simulink library "bcm"  (R2021b)
settings: Solver=VariableStepAuto  StartTime=0.0  StopTime=10.0  RelTol=1e-3
undefined symbols (not defined in the file or in its folder): KBCM_ShowUPT_cnt
libraries: simulink x33
(part 2 of 2)

== stateflow chart bcm/BCM/BCM/ExteriorLight/Chart1 ==
  state FollowMeSW [parallel]
    settings: executionOrder=1
    state sRelease
    state sPress
    (default) -> sRelease
    sRelease -> sPress : [VINP_FollowMeSW_flg==1]/{AutoCut.eFollow;}
    sPress -> sRelease : [VINP_FollowMeSW_flg==0]
  state RFogLamp [parallel]
    settings: executionOrder=2
    state sON
      en:VBCM_RrFogLamp_flg=1;
    state sOFF
      en:VBCM_RrFogLamp_flg=0;
    (default) -> RFogLamp.sOFF
    RFogLamp.sOFF -> RFogLamp.sON : [VPMM_PwrSta_enum>3&&....
        | VINP_RFogLampSW_flg==1&&....
        | VBCM_LBeam_flg==1]
    RFogLamp.sON -> RFogLamp.sOFF : [VPMM_PwrSta_enum<=3||....
        | VINP_RFogLampSW_flg==0||....
        | VBCM_LBeam_flg==0]
  state DRL [parallel]
    settings: executionOrder=3
    state sOFF
      en:VBCM_LDRL_flg=0;
      VBCM_RDRL_flg=0;
    state DRL_Opearting
      state sDebounce
      state sON
        en:VBCM_LDRL_flg=1;
        VBCM_RDRL_flg=1;
      note: 300 ms
      state TurnLeft
        en:VBCM_LDRL_flg=0;
        VBCM_RDRL_flg=1;
      state TurnRight
        en:VBCM_LDRL_flg=1;
        VBCM_RDRL_flg=0;
      sDebounce -> (junction 119) : [after(30,tick)]
      (junction 119) -> DRL.DRL_Opearting.sON [order 1] : [VBCM_OutMode_enum==0]
      (junction 119) -> (junction 120) [order 2]
      DRL.DRL_Opearting.sON -> TurnLeft [order 1] : [VBCM_OutMode_enum==1]
      TurnLeft -> DRL.DRL_Opearting.sON [order 1] : [VBCM_OutMode_enum==0]
      TurnRight -> DRL.DRL_Opearting.sON [order 2] : [VBCM_OutMode_enum==0]
      DRL.DRL_Opearting.sON -> TurnRight [order 2] : [VBCM_OutMode_enum==2]
      (junction 120) -> TurnLeft [order 1] : [VBCM_OutMode_enum==1]
      (junction 120) -> (junction 121) [order 2]
      TurnRight -> TurnLeft [order 1] : [VBCM_OutMode_enum==1]
      TurnLeft -> TurnRight [order 2] : [VBCM_OutMode_enum==2]
      (junction 121) -> TurnRight
    (default) -> DRL.sOFF
    DRL.sOFF -> sDebounce : [VPMM_PwrSta_enum>3 &&...
        | !VBCM_PosLamp_flg&&...
        | VBCM_OutMode_enum < 3]
    DRL_Opearting -> DRL.sOFF : [VPMM_PwrSta_enum<=3 ||...
        | VBCM_PosLamp_flg ||...
        | VBCM_OutMode_enum >= 3]
  state sBrakeLamp [parallel]
    settings: executionOrder=4
    state sON
      en:VBCM_BrakeLamp_flg=1;
    state sOFF
      en:VBCM_BrakeLamp_flg=0;
    (default) -> sBrakeLamp.sOFF
    sBrakeLamp.sOFF -> sBrakeLamp.sON : [VINP_BrakeSWGPIO_flg==1 || VTQD_ReBrakeLPReq_flg==1 || VINP_ActBrkLampSta_flg==1]
    sBrakeLamp.sON -> sBrakeLamp.sOFF : [VINP_BrakeSWGPIO_flg==0 && VTQD_ReBrakeLPReq_flg==0 && VINP_ActBrkLampSta_flg==0]
  state sReverseLamp [parallel]
    settings: executionOrder=5
    state sON
      en:VBCM_ReverseLamp_flg=1;
    state sOFF
      en:VBCM_ReverseLamp_flg=0;
    (default) -> sReverseLamp.sOFF
    sReverseLamp.sOFF -> sReverseLamp.sON : [VPMM_PwrSta_enum>3&&VTQD_ShiftGearPosn_enum==7]
    sReverseLamp.sON -> sReverseLamp.sOFF : [VPMM_PwrSta_enum<=3||VTQD_ShiftGearPosn_enum!=7]
  state sATCtrl [parallel]
    settings: executionOrder=6
    state StandBy
    state Lock
      en:send(AutoCut.eLock);
    state Unlock
      en:send(AutoCut.eUnlock);
    (default) -> StandBy
    StandBy -> Lock [order 1] : [VINP_PDKeyAreaLockUnlock_enum==1]
    Lock -> StandBy : [VINP_PDKeyAreaLockUnlock_enum!=1]
    StandBy -> sATCtrl.Unlock [order 2] : [VINP_PDKeyAreaLockUnlock_enum==2]
    sATCtrl.Unlock -> StandBy : [VINP_PDKeyAreaLockUnlock_enum!=2]
  state PositionLamp [parallel]
    settings: executionOrder=7
    state sPositionLamp
      en:VBCM_PosLamp_flg=1;
    state sOFF
      en:VBCM_PosLamp_flg=0;
    (default) -> PositionLamp.sOFF
    (junction 94) -> sPositionLamp [order 1] : [VINP_HeadLampSW_enum==1||VINP_HeadLampSW_enum==2]
    PositionLamp.sOFF -> (junction 94) [order 1] : [!VBCM_AutoCut_flg]
    (junction 94) -> (junction 95) [order 2]
    (junction 95) -> sPositionLamp [order 1] : [VPMM_PwrSta_enum>3&&VINP_HeadLampSW_enum==0&&VINP_RLSLampSta_flg]
    (junction 95) -> (junction 96) [order 2]
    (junction 96) -> sPositionLamp : [VBCM_FollowMe_flg]
    PositionLamp.sOFF -> sPositionLamp [order 2] : [VBCM_showup_flg]
    (junction 97) -> PositionLamp.sOFF : [!VBCM_FollowMe_flg&&(VINP_HeadLampSW_enum==3||....
        | (VINP_HeadLampSW_enum==0&&(VPMM_PwrSta_enum<=3||!VINP_RLSLampSta_flg)))]
    (junction 98) -> (junction 97) [order 2]
    (junction 98) -> PositionLamp.sOFF [order 1] : [VBCM_AutoCut_flg]
    sPositionLamp -> (junction 98) : [!VBCM_showup_flg]
  state AutoCut [parallel]
    settings: executionOrder=8
    state FollowMeHome
      en:
      VBCM_FollowMe_flg=1;
      VBCM_AutoCut_flg=0;
      VBCM_showup_flg=0;
      ex:
      VBCM_FollowMe_flg=0;
    state Normal
      state sNormal
        en:VBCM_AutoCut_flg=0;
        VBCM_showup_flg=0;
      state AutoCutDetect
      note: 40 sec
      state Unlock
        en:VBCM_AutoCut_flg=1;
        VBCM_showup_flg=1;
        note: 30 sec
      state AutoCut
        en:VBCM_AutoCut_flg=1;
        VBCM_showup_flg=0;
        VBCM_FollowMe_flg=0;
      sNormal -> AutoCutDetect : [VPMM_PwrSta_enum<=3&&(VINP_HeadLampSW_enum!=3)]
      (junction 64) -> sNormal : [VPMM_PwrSta_enum>3||VINP_HeadLampSW_enum==3]
      AutoCutDetect -> (junction 64) [order 1]
      AutoCut.Normal.AutoCut -> (junction 64)
      AutoCutDetect -> AutoCut.Normal.AutoCut [order 2] : eLock
      AutoCutDetect -> AutoCut.Normal.AutoCut [order 3] : [after(4000,tick)]
      AutoCut.Normal.Unlock -> sNormal [order 2] : [VPMM_PwrSta_enum>3]
      (default) -> AutoCut.Normal.AutoCut
      AutoCut.Normal.Unlock -> AutoCut.Normal.AutoCut [order 1] : eLock
      AutoCut.Normal.Unlock -> AutoCut.Normal.AutoCut [order 3] : [after(3000,tick)]
      Normal -> AutoCut.Normal.Unlock [order 1] : eUnlock[VPMM_PwrSta_enum<=3]
    note: 4000
    note: 40 sec
    (default) -> Normal
    Normal -> FollowMeHome [order 1] : eFollow[VPMM_PwrSta_enum<=3]
    FollowMeHome -> sNormal [order 2] : eFollow
    FollowMeHome -> sNormal [order 3] : [VPMM_PwrSta_enum>3]
    (junction 52) -> sNormal [order 1] : [VPMM_PwrSta_enum>3||...
        |  VINP_HeadLampSW_enum==3]
    FollowMeHome -> (junction 52) [order 1] : [after(4000,tick)]
    (junction 52) -> (junction 53) [order 2]
    (junction 53) -> AutoCut.Normal.AutoCut
  state LowBeam [parallel]
    settings: executionOrder=9
    state sLBeam
      en:VBCM_LBeam_flg=1;
    state sOFF
      en:VBCM_LBeam_flg=0;
    (default) -> LowBeam.sOFF
    (junction 8) -> sLBeam [order 1] : [VBCM_HBeam_flg]
    LowBeam.sOFF -> (junction 8) [order 1] : [!VBCM_AutoCut_flg]
    (junction 8) -> (junction 9) [order 2]
    (junction 9) -> sLBeam [order 1] : [VINP_HeadLampSW_enum==2]
    (junction 9) -> (junction 10) [order 2]
    (junction 10) -> sLBeam [order 1] : [VPMM_PwrSta_enum>3&&VINP_HeadLampSW_enum==0&&VINP_RLSLampSta_flg]
    (junction 10) -> (junction 11) [order 2]
    (junction 11) -> sLBeam : [VBCM_FollowMe_flg]
    LowBeam.sOFF -> sLBeam [order 2] : [VBCM_showup_flg]
    (junction 12) -> LowBeam.sOFF [order 1] : [VBCM_AutoCut_flg]
    sLBeam -> (junction 12) : [!VBCM_showup_flg]
    (junction 12) -> (junction 13) [order 2]
    (junction 13) -> LowBeam.sOFF : [!VBCM_FollowMe_flg&&!VBCM_HBeam_flg&&VINP_HeadLampSW_enum!=2&&....
        | (VINP_HeadLampSW_enum!=0||!VINP_RLSLampSta_flg||VPMM_PwrSta_enum<=3)]
  state HighBeam [parallel]
    settings: executionOrder=10
    state sHBeam
      en:VBCM_HBeam_flg=1;
    state sOFF
      en:VBCM_HBeam_flg=0;
    (default) -> HighBeam.sOFF
    HighBeam.sOFF -> (junction 140) : [!VBCM_AutoCut_flg]
    (junction 140) -> sHBeam [order 1] : [VINP_CSWPassSWSta_flg]
    (junction 140) -> (junction 141) [order 2]
    (junction 141) -> (junction 142) : [VINP_CSWDimSw_flg]
    (junction 142) -> sHBeam [order 1] : [VINP_HeadLampSW_enum==2]
    (junction 142) -> (junction 143) [order 2]
    (junction 143) -> sHBeam : [VINP_HeadLampSW_enum==0&&VINP_RLSLampSta_flg==1&&VPMM_PwrSta_enum>3]
    sHBeam -> HighBeam.sOFF [order 1] : [VBCM_AutoCut_flg]
    (junction 144) -> HighBeam.sOFF [order 1] : [!VINP_CSWDimSw_flg]
    sHBeam -> (junction 144) [order 2] : [!VINP_CSWPassSWSta_flg]
    (junction 144) -> (junction 146) [order 2]
    (junction 145) -> HighBeam.sOFF [order 1] : [VINP_HeadLampSW_enum!=0]
    (junction 146) -> (junction 145) : [VINP_HeadLampSW_enum!=2]
    (junction 145) -> (junction 147) [order 2]
    (junction 147) -> HighBeam.sOFF : [VINP_RLSLampSta_flg==0||VPMM_PwrSta_enum<=3]
  data: VBCM_OutMode_enum input uint8; VINP_ActBrkLampSta_flg input boolean; VINP_BrakeSWGPIO_flg input boolean; VINP_CSWDimSw_flg input boolean; VINP_CSWPassSWSta_flg input boolean; VINP_FollowMeSW_flg input boolean; VINP_HeadLampSW_enum input uint8; VINP_PDKeyAreaLockUnlock_enum input uint8; VINP_RFogLampSW_flg input boolean; VINP_RLSLampSta_flg input boolean; VPMM_PwrSta_enum input uint8; VTQD_ReBrakeLPReq_flg input boolean; VTQD_ShiftGearPosn_enum input uint8; VBCM_BrakeLamp_flg output boolean; VBCM_LDRL_flg output boolean; VBCM_RDRL_flg output boolean; VBCM_ReverseLamp_flg output boolean; VBCM_RrFogLamp_flg output boolean; VBCM_AutoCut_flg local boolean; VBCM_FollowMe_flg local boolean; VBCM_HBeam_flg output boolean; VBCM_LBeam_flg output boolean; VBCM_PosLamp_flg output boolean; VBCM_showup_flg local boolean
  events: eLock local FUNCTION_CALL_EVENT; eUnlock local FUNCTION_CALL_EVENT; eFollow local FUNCTION_CALL_EVENT

== stateflow chart bcm/BCM/BCM/FlasherSignal/Chart ==
  settings: updateMethod=DISCRETE
  state sModeSelect [parallel]
    settings: executionOrder=2  description=This state models the modes of a door sensor and implements logic to respond when that sensor is producing a signal.
    state sStandBy
    (default) -> sStandBy
      settings: description=On the first sample call the door mode is set to active.
    sStandBy -> (junction 1969)
    (junction 1971) -> sStandBy
    (junction 1969) -> (junction 1971) [order 1] : [InputMode==4||InputMode==5]
    (junction 1969) -> (junction 1871) [order 2]
    (junction 1873) -> (junction 1971)
    (junction 1871) -> (junction 1873) [order 1] : [PwrSta>3&&ESS_Active==1]{InputMode=7;}
    (junction 1871) -> (junction 1987) [order 2]
    (junction 1989) -> (junction 1873)
    (junction 1987) -> (junction 1989) [order 1] : [HazardSW==1]{InputMode=3;}
    (junction 1987) -> (junction 1876) [order 2]
    (junction 1878) -> (junction 1989)
    (junction 1876) -> (junction 1878) [order 1] : [PwrSta>3&&CSW_TurnSw_Sta==1]{InputMode=1;}
    (junction 1876) -> (junction 1882) [order 2]
    (junction 1884) -> (junction 1878)
    (junction 1882) -> (junction 1884) [order 1] : [PwrSta>3&&CSW_TurnSw_Sta==2]{InputMode=2;}
    (junction 1882) -> (junction 1887) [order 2]
    (junction 1889) -> (junction 1884)
    (junction 1887) -> (junction 1889) : /{InputMode=0;}
  state HazardSW [parallel]
    settings: executionOrder=1
    state Normal
      state sHAZARDOFF
      state Press
      state sHAZARDON
      (default) -> sHAZARDOFF
      sHAZARDOFF -> Press : [HazardSWSta==1]/{HazardSW=1;}
      (junction 1864) -> sHAZARDOFF [order 1] : [HazardSW==0]
      Press -> (junction 1864) : [HazardSWSta==0]
      (junction 1864) -> sHAZARDON [order 2]
      sHAZARDON -> Press : [HazardSWSta==1]{HazardSW=0;}
    (default) -> Normal
  state sATCtrl [parallel]
    settings: executionOrder=4
    state StandBy
    state Lock
      en:InputMode=4;
    state Unlock
      en:InputMode=5;
    (default) -> StandBy
    StandBy -> Lock [order 1] : [VINP_PDKeyAreaLockUnlock_enum==1]
    Lock -> StandBy : [VINP_PDKeyAreaLockUnlock_enum!=1]
    StandBy -> Unlock [order 2] : [VINP_PDKeyAreaLockUnlock_enum==2 ||VBCM_FindCar_flg ]
    Unlock -> StandBy : [VINP_PDKeyAreaLockUnlock_enum!=2&&!VBCM_FindCar_flg]
  state Main [parallel]
    settings: executionOrder=3
    state sUnLockOFF1
      en:InputMode=0;
    state sUnLockOFF
      en:LTurnLP=0;
      RTurnLP=0;
      FlashCount=FlashCount-1;
    state sHazardOFF
      en:LTurnLP=0;
      RTurnLP=0;
    state sESSOFF
      en:LTurnLP=0;
      RTurnLP=0;
    state sLockOFF
      en:LTurnLP=0;
      RTurnLP=0;
      InputMode=0;
    state sAlarmOFF
      en:LTurnLP=0;
      RTurnLP=0;
    note: 500 ms
    note: 600 ms
    note: 500 ms
    note: 460 ms
    note: 460 ms
    state sHazardON
      en:LTurnLP=1;
      RTurnLP=1;
      FDC_BCM_BBuzzer_Cmd=1;
      ex:FDC_BCM_BBuzzer_Cmd=0;
    state sLock
      en:LTurnLP=1;
      RTurnLP=1;
    state sAlarm
      en:LTurnLP=1;
      RTurnLP=1;
    state sESSON
      en:LTurnLP=1;
      RTurnLP=1;
      FDC_BCM_BBuzzer_Cmd=1;
      ex:FDC_BCM_BBuzzer_Cmd=0;
    state sUnlock
      en:LTurnLP=1;
      RTurnLP=1;
    state sWait
      en:LTurnLP=0;RTurnLP=0;
    note: 120 ms
    state sOFF
      en:LTurnLP=0;RTurnLP=0;
    state sLeftON
      en:LTurnLP=1;
      RTurnLP=0;
      FDC_BCM_BBuzzer_Cmd=1;
      ex:FDC_BCM_BBuzzer_Cmd=0;
    state sRightON
      en:LTurnLP=0;
      RTurnLP=1;
      FDC_BCM_BBuzzer_Cmd=1;
      ex:FDC_BCM_BBuzzer_Cmd=0;
    state sOFF1
      en:LTurnLP=0;
      RTurnLP=0;
    Main -> sWait : [OutMode!=InputMode]
        | {OutMode=InputMode;}
    sUnLockOFF -> sUnLockOFF1 [order 1] : [FlashCount==0]
    sLock -> sLockOFF : [after(50,tick)]
    sAlarm -> sAlarmOFF : [after(50,tick)]
    sAlarmOFF -> sAlarm : [after(50,tick)]
    sHazardON -> sHazardOFF : [after(46,tick)]
    sHazardOFF -> sHazardON : [after(46,tick)]
    sESSON -> sESSOFF : [after(13,tick)]
    sESSOFF -> sESSON : [after(12,tick)]
    sUnlock -> sUnLockOFF : [after(20,tick)]
    sUnLockOFF -> sUnlock [order 2] : [after(60,tick)]
    sOFF -> sUnlock [order 8] : [InputMode==9]....
        | {FlashCount=2;}
    sOFF -> sUnlock [order 3] : [OutMode==5]....
        | {FlashCount=3;}
    sOFF -> sLock [order 1] : [OutMode==4]
    sOFF -> sAlarm [order 4] : [OutMode==6]
    (default) -> sOFF
    sWait -> sOFF : [after(12,tick)]
    sOFF -> sESSON [order 2] : [OutMode==7]
    sOFF -> sHazardON [order 7] : [OutMode==3]
    sOFF -> sLeftON [order 5] : [OutMode==1]
    sOFF -> sRightON [order 6] : [OutMode==2]
    (junction 1940) -> sLeftON [order 1] : [OutMode==1]
    (junction 1940) -> sRightON [order 2]
    sOFF1 -> (junction 1940) : [after(46,tick)]
    sLeftON -> sOFF1 : [after(46,tick)]
    sRightON -> sOFF1 : [after(46,tick)]
  data: VINP_PDKeyAreaLockUnlock_enum input uint8 [0..2]; PwrSta input uint8 [0..5]; HazardSWSta input boolean [0..1]; CSW_TurnSw_Sta input uint8 [0..3]; HazardSW output boolean =0; LTurnLP output boolean; RTurnLP output boolean; InputMode local uint8; FlashCount local uint8; OutMode output uint8; ESS_Active input boolean; VBCM_FindCar_flg input boolean; FDC_BCM_BBuzzer_Cmd output boolean

== stateflow chart bcm/BCM/BCM/WasherWiper/Chart ==
  settings: sampleTime=StepSize
  state sWasher [parallel]
    settings: executionOrder=2  description=This state models the modes of a door sensor and implements logic to respond when that sensor is producing a signal.
    state sOFF
      en:WasherControl=0;
    state sFWasher
      note: 300 ms
      state sFrontWasher
        en:WasherControl=1;
      state sFrontWasher1
        en:WasherControl=1;
        FWasherCount=3;
      sFrontWasher -> sFrontWasher1 : [after(30,tick)]
    (default) -> sWasher.sOFF
      settings: description=On the first sample call the door mode is set to active.
    sFWasher -> sWasher.sOFF : [PwrSta<=3||CSW_FWasSw_Sta!=1]
    sWasher.sOFF -> sFrontWasher : [PwrSta>3&&CSW_FWasSw_Sta==1]
  state FrontWiper [parallel]
    settings: executionOrder=1
    state Wiping
      state sHIGHSPEED
        en:FWiperH=1;FWiperL=0;
      state sLOWSPEED
        en:FWiperH=0;FWiperL=1;
      Wiping -> (junction 1869) [order 1]
      (junction 1869) -> sHIGHSPEED [order 1] : [CSW_FWipSw_Sta==3]
      (junction 1869) -> (junction 1870) [order 2]
      (junction 1870) -> (junction 1871) [order 1] : [CSW_FWipSw_Sta==1]
      (junction 1871) -> sHIGHSPEED [order 1] : [ RLS_RainSnrWiperCmd==3]
      (junction 1870) -> (junction 1873) [order 2]
      (junction 1871) -> (junction 1985) [order 2]
      (junction 1985) -> sLOWSPEED : [RLS_RainSnrWiperCmd==2]
      (junction 1873) -> sLOWSPEED [order 1] : [CSW_FWipSw_Sta==2]
      (junction 1873) -> (junction 1874) [order 2]
      (junction 1874) -> sLOWSPEED [order 1] : [CSW_FWasSw_Sta==2]
      (junction 1874) -> (junction 1875) [order 2]
      (junction 1875) -> (junction 1876) [order 1] : [FWasherCount>0]
      (junction 1876) -> sLOWSPEED [order 1] : [VINP_FWiperProtection_flg == 0]
      (junction 1876) -> (junction 1877) [order 2]
    state sOFF
      en:FWiperH=0;FWiperL=0;
    (default) -> FrontWiper.sOFF
    FrontWiper.sOFF -> (junction 1869) : [PwrSta>3]
    Wiping -> FrontWiper.sOFF [order 1] : [PwrSta<=3]
    (junction 1875) -> FrontWiper.sOFF [order 2]
    (junction 1877) -> FrontWiper.sOFF : {FWasherCount = 0;}
  state sFWasherWipingMode [parallel]
    settings: executionOrder=3
    state sOFF
      en:FWasherCount=0;
    state sON
      state sClean
        state sNotPark
          en:FWasherCount=FWasherCount-1;
        state sPark1
        (junction 1967) -> sNotPark [order 1] : [FWiperAS==1]
        sNotPark -> sPark1 : [FWiperAS==0]
        sPark1 -> sNotPark : [FWiperAS==1]
        (junction 1967) -> sPark1 [order 2]
      state ON
      ON -> (junction 1962) : [WasherControl!=1]
      (junction 1962) -> (junction 1967) [order 2]
      sClean -> ON [order 1] : [WasherControl==1]
    (default) -> sFWasherWipingMode.sOFF
    sFWasherWipingMode.sOFF -> ON : [PwrSta>3&&WasherControl==1]
    (junction 1962) -> sFWasherWipingMode.sOFF [order 1] : [FWasherCount == 0]
    sClean -> sFWasherWipingMode.sOFF [order 2] : [FWasherCount == 0]
    sON -> sFWasherWipingMode.sOFF : [PwrSta <= 3]
  data: CSW_FWasSw_Sta input uint8 [0..3]; CSW_FWipSw_Sta input uint8 [0..7]; RLS_RainSnrWiperCmd input uint8 [0..7]; FWiperAS input boolean; FWiperL output boolean; FWiperH output boolean; FWasherCount local uint8; RWasherCount local uint8; WasherControl output uint8; PwrSta input uint8 [0..5]; VINP_FWiperProtection_flg input boolean
